simulink subsystem "Receber_Dados_do_MCU"  (R2023b)
settings: Solver=VariableStepAuto  StartTime=0.0  StopTime=10.0  RelTol=1e-3
libraries: etargetslib x1
settings Model: Creator=Ricardo  LastModifiedBy=Ricardo

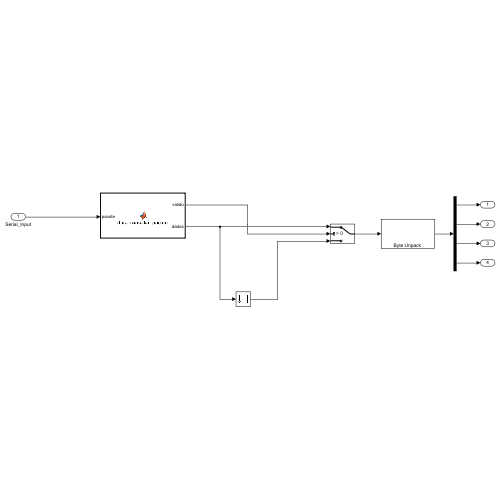
[thumbnail: Simulink's stored preview of the top-level diagram]
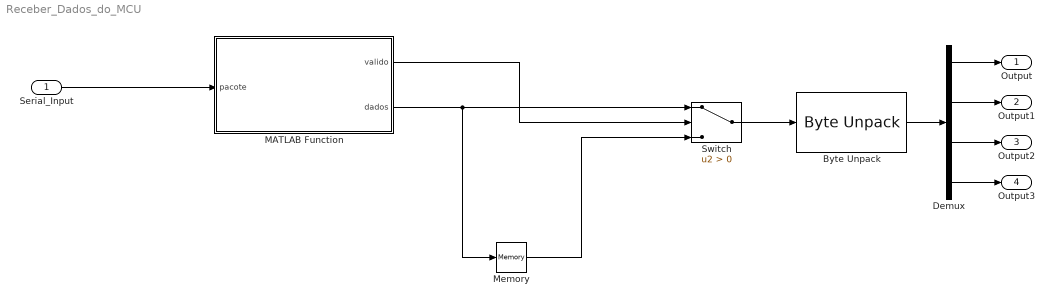
== system Receber_Dados_do_MCU ==
  Serial_Input : Inport
  Byte Unpack : etargetslib/Byte Unpack  dimensions={[1]}  datatypes={'double'}  byteAlign=1
      settings: LibrarySourceBlock=embeddedtargetslib/Host Communication/Byte Unpack
  Demux : Demux
  MATLAB Function : MATLAB Function  TreatAsAtomicUnit=on
  Memory : Memory
  Switch : Switch  Criteria=u2 > Threshold  SaturateOnIntegerOverflow=off  InputSameDT=off
  Output : Outport
  Output1 : Outport  Port=2
  Output2 : Outport  Port=3
  Output3 : Outport  Port=4
  wires:
  Serial_Input/1 -> MATLAB Function/1(pacote)
  MATLAB Function/1(valido) -> Switch/2
  MATLAB Function/2(dados) -> Memory/1, Switch/1
  Memory/1 -> Switch/3
  Switch/1 -> Byte Unpack/1
  Byte Unpack/1 -> Demux/1
  Demux/1 -> Output/1
  Demux/2 -> Output1/1
  Demux/3 -> Output2/1
  Demux/4 -> Output3/1

== matlab function Receber_Dados_do_MCU/MATLAB Function ==
  data: pacote input; valido output; dados output
function [valido, dados] = desempacotar_pacote(pacote)
    START_BYTE = uint8(170);  % 0xAA
    PACKET_TYPE = uint8(2);   % 0x02 para saída
    END_BYTE = uint8(85);     % 0x55
    
    valido = false;
    dados = zeros(4, 1);
    
    if pacote(1) == START_BYTE && pacote(end) == END_BYTE && pacote(2) == PACKET_TYPE
        comprimento = pacote(3);
        dados_bytes = pacote(4:end-2);
        checksum_recebido = pacote(end-1);
        
        if length(dados_bytes) == comprimento
            checksum_calculado = uint8(mod(sum(pacote(2:end-2)), 256));
            if checksum_calculado == checksum_recebido
                dados = typecast(dados_bytes, 'double');
                valido = true;
            end
        end
    end
end
